simulink subsystem "EKF_old_daniele"  (R2024a)
settings: Solver=VariableStepAuto  StartTime=0.0  StopTime=10.0  RelTol=1e-3
undefined symbols (not defined in the file): R_KF
settings Model: Creator=Bocchio  LastModifiedBy=cianc

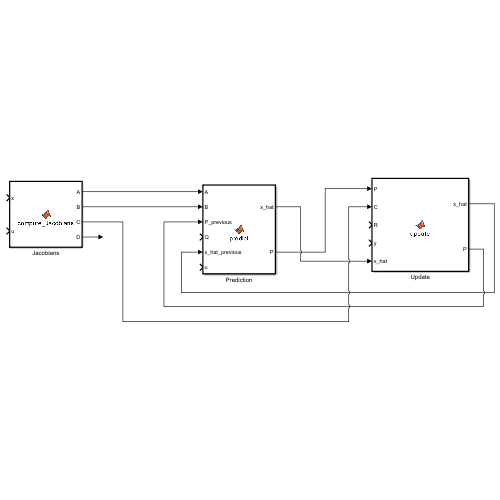
[thumbnail: Simulink's stored preview of the top-level diagram]
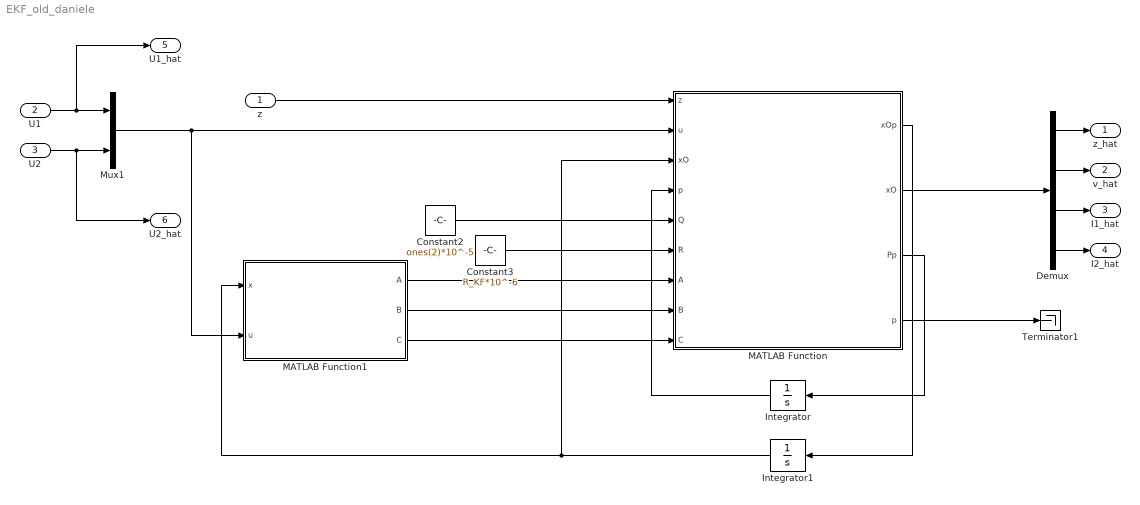
== system EKF_old_daniele ==
  z : Inport
  U1 : Inport  Port=2
  U2 : Inport  Port=3
  Constant2 : Constant  Value=ones(2)*10^-5
  Constant3 : Constant  Value=R_KF*10^-6
  Demux : Demux
  Integrator : Integrator  InitialCondition=ones(16,1)*10^-7
  Integrator1 : Integrator  InitialCondition=[0.01,0,0.835,0]'
  MATLAB Function : MATLAB Function  TreatAsAtomicUnit=on
  MATLAB Function1 : MATLAB Function  TreatAsAtomicUnit=on
  Mux1 : Mux  Inputs=2
  Terminator1 : Terminator
  z_hat : Outport
  v_hat : Outport  Port=2
  I1_hat : Outport  Port=3
  I2_hat : Outport  Port=4
  U1_hat : Outport  Port=5
  U2_hat : Outport  Port=6
  wires:
  Demux/1 -> z_hat/1
  MATLAB Function1/3(C) -> MATLAB Function/9(C)
  Integrator1/1 -> MATLAB Function/3("xO "), MATLAB Function1/1(x)
  Mux1/1 -> MATLAB Function/2(u), MATLAB Function1/2(u)
  z/1 -> MATLAB Function/1(z)
  MATLAB Function1/2(B) -> MATLAB Function/8(B)
  U1/1 -> Mux1/1, U1_hat/1
  MATLAB Function/2(xO) -> Demux/1
  MATLAB Function/3(Pp) -> Integrator/1
  Integrator/1 -> MATLAB Function/4("p ")
  Constant2/1 -> MATLAB Function/5(Q)
  MATLAB Function1/1(A) -> MATLAB Function/7(A)
  MATLAB Function/4(p) -> Terminator1/1
  MATLAB Function/1(xOp) -> Integrator1/1
  Constant3/1 -> MATLAB Function/6(R)
  U2/1 -> Mux1/2, U2_hat/1
  Demux/2 -> v_hat/1
  Demux/3 -> I1_hat/1
  Demux/4 -> I2_hat/1

== matlab function EKF_old_daniele/MATLAB Function ==
  data: z input; u input; xOp output; xO input; xO output; Pp output; p output; p input; Q input; R input; A input; B input; C input
function [xOp,xO,Pp,p]  = obs(z,u,xO,p,Q,R,A,B,C)

Nstates = size(xO,1);
Pp = zeros(Nstates^2,1);

%% Differential Riccati Equation - Computation of the gain matrix K

% transformation vector -> matrix
P = zeros(Nstates,Nstates);
P(1:end) = p(1:end,1);

% DRE
Out = (A*P + P*A' + B*Q*B' - P*C'*R^-1*C*P);

K = P*C'*inv(R);

% transformation matrix -> vector
Pp(1:end,1) = Out(1:end)';

%% State estimate

xOp = A * xO + B * u;
xOp = xOp + K*(z - C*xO);

== matlab function EKF_old_daniele/MATLAB Function1 ==
  settings: updateMethod=DISCRETE
  data: x input; A output; B output; C output; u input
function [A, B, C] = compute_Jacobians(x,u)

%% U to V
measurements.pwm = 0:0.1:1;
measurements.voltage = [0.043 0.613 1.768 2.93 4.10 5.26 6.43 7.59 8.80 9.96 11.06];

p = polyfit(measurements.pwm(2:end), measurements.voltage(2:end), 1);

voltage_min = min(measurements.voltage);
PWM_min = (voltage_min - p(2)) / p(1);

voltage = @(PWM) ...
    (PWM < PWM_min) .* (voltage_min) + ...
    (PWM >= PWM_min) .* (p(1) * PWM + p(2));
%% 
L1 = 0;
L2 = 0;
dL1dx = 0;
dL2dx = 0;
dL1ddx = 0;
dL2ddx = 0;
A = zeros(4);
B = zeros(4,2);
C = zeros(1,4);
%% Parameters

% Physical constants
g   = 9.81; %[m/s^2]

% Structure
H = 98.00 * 1e-3; %[m]

% Ball/object
m = 60.54 * 1e-3;   %[kg]
r = 61.25/2 * 1e-3; %[m]

%% Drag related coefficients
rho = 1.21; %[kg/m^3]
Cd  = 0.45; %[Ns/m]

%% Current model
V1min = 4.300000e-02; %[V]
V2min = 4.300000e-02; %[V]
I1min = 2.383122e-02; %[A]
I2min = 2.591441e-02; %[A]
k1 = +1.165800e+01; %[V/MU]
k2 = +1.165800e+01; %[V/MU]
c1 = -5.608000e-01; %[V]
c2 = -5.608000e-01; %[V]

%% Inductances
% L(z, I) = L0 + Lz * exp(-az * z) + LI * atan(aI * I - bI);

% Static
L10 = 6.122809e-02; %[H]
L20 = 6.122809e-02; %[H]

% Position z
a1z = 1.837302e+02; %[1/m]
a2z = 1.837302e+02; %[1/m]
L1z = 3.438228e-02; %[H]
L2z = 3.438228e-02; %[H]

% Current I
a1I = 4.759750e+00; %[]
a2I = 4.759750e+00; %[]
b1I = 6.704755e-01; %[A]
b2I = 6.704755e-01; %[A]
L1I = 3.831209e-02; %[H]
L2I = 3.831209e-02; %[H]

%% Resistances
% R() = R0

% Static
R10 = 4.17; %[ohm]
R20 = 4.20; %[ohm]

%%

L1 = @(x, I) L10 + L1z * exp(-a1z*x) + L1I * atan(a1I * I - b1I);
L2 = @(x, I) L20 + L2z * exp(-a2z*(H - 2*r - x)) + L2I * atan(a2I * I - b2I);
dL1dx = @(x) -a1z*L1z * exp(-a1z*x);
dL2dx = @(x) +a2z*L2z * exp(-a2z*(H - 2*r - x));
dL1ddx = @(x) +a1z^2*L1z * exp(-a1z*x);
dL2ddx = @(x) +a2z^2*L2z * exp(-a2z*(H - 2*r - x));

% A coefficients
a11 = 0;
a12 = 1;
a13 = 0;
a14 = 0;

a21 = 1 / m * (1/2 * dL1ddx(x(1)) * x(3)^2 + 1/2 * dL2ddx(x(1)) * x(4)^2);
a22 = 0;
a23 = 1/m * dL1dx(x(1)) * x(3);
a24 = 1/m * dL2dx(x(1)) * x(4);

a31 = -1 / L1(x(1), x(3))^2 * dL1dx(x(1)) * (-R10 * x(3) + U_to_V(u(1)));
a32 = 0;
a33 = 1 / L1(x(1), x(3)) * (-R10);
a34 = 0;

a41 = -1 / L2(x(1), x(4))^2 * dL2dx(x(1)) * (-R20 * x(4) + U_to_V(u(2)));
a42 = 0;
a43 = 0;
a44 = 1 / L2(x(1), x(4)) * (-R20);

% B coefficients
b11 = 0;
b12 = 0;
b21 = 0;
b22 = 0;
b31 = 1 / L1(x(1), x(3)) * k1;
b32 = 0;
b41 = 0;
b42 = 1 / L2(x(1), x(4)) * k2;

% C coefficients
c1 = 1;
c2 = 0;
c3 = 0;
c4 = 0;

% State matrices
A = [
    a11 a12 a13 a14;
    a21 a22 a23 a24;
    a31 a32 a33 a34;
    a41 a42 a43 a44
    ];

B = [
    b11 b12;
    b21 b22;
    b31 b32;
    b41 b42
    ];

C = [c1 c2 c3 c4];

end
